simulink model "untitled"  (R2019a)
settings: Solver=VariableStepAuto  StartTime=0.0  StopTime=1  RelTol=1e-3
values from neighbouring files (symbols this model uses):
  Ts_Control = 5.0000e-05    (= 5e-05)    [Sec_Impedance.m]
  Ts_Power = 5.0000e-05    (= 5e-05)    [Sec_Impedance.m]
undefined symbols (not defined in the file or in its folder): D1, Delta, Ion, Lithium
libraries: powerlib x152, powerlib_meascontrol x65, simulink x14, electricdrivelib x12, simulink_extras x12
(part 1 of 5)
settings Model: SimulationMode=accelerator  Creator=ASUS  LastModifiedBy=ASUS

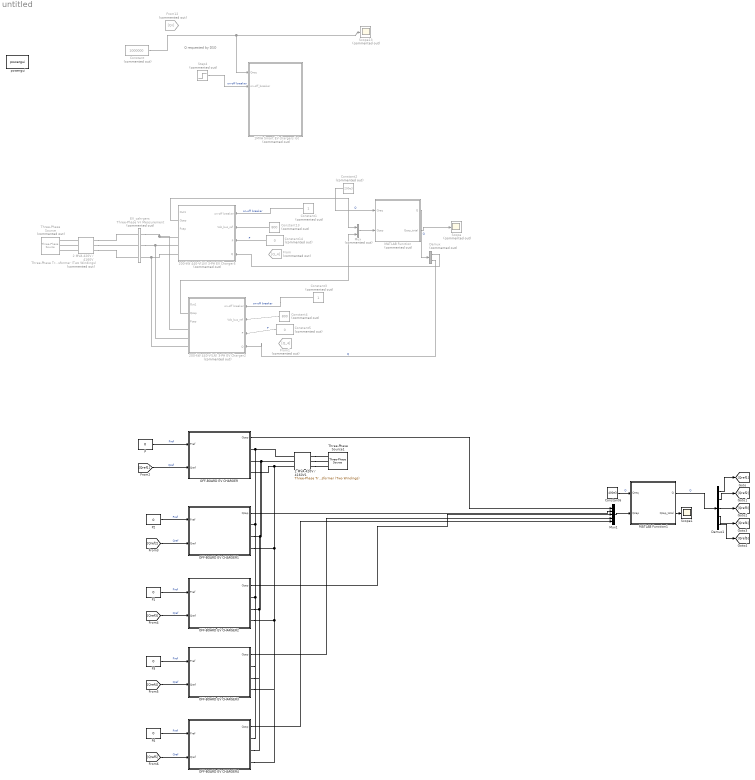
== system untitled ==
  note: Q requested by DSO
  1MVA Smart EV chargers lot : Subsystem  Commented=on
  2 MVA 420V / 4160V : powerlib/Elements/Three-Phase Transformer (Two Windings)  Commented=on  Winding1Connection=Delta (D1)  Winding2Connection=Yg  CoreType=Three single-phase transformers  SetSaturation=off  Hysteresis=off  DataFile='hysteresis'  SetInitialFlux=off  Measurements=None  UNITS=pu  NominalPower=[5e6 , 60 ]  Winding1=[ 4160 , 0.001 , 0.03 ]  Winding2=[ 420 , 0.001 , 0.03 ]  Rm=500  Lm=500  L0=0.5  Saturation=[ 0,0 ; 0.0024,1.2 ; 1.0,1.52 ]  InitialFluxes=[0.79999 -0.79999 0.7]  BreakLoop=off  DiscreteSolver=Trapezoidal iterative  DataType=off  TransfoNumber=0
      settings: SourceProductName=Simscape Electrical
  2 MVA 420V / 4160V1 : powerlib/Elements/Three-Phase Transformer (Two Windings)  Winding1Connection=Delta (D1)  Winding2Connection=Yg  CoreType=Three single-phase transformers  SetSaturation=off  Hysteresis=off  DataFile='hysteresis'  SetInitialFlux=off  Measurements=None  UNITS=pu  NominalPower=[5e6 , 60 ]  Winding1=[ 4160 , 0.001 , 0.03 ]  Winding2=[ 420 , 0.001 , 0.03 ]  Rm=500  Lm=500  L0=0.5  Saturation=[ 0,0 ; 0.0024,1.2 ; 1.0,1.52 ]  InitialFluxes=[0.79999 -0.79999 0.7]  BreakLoop=off  DiscreteSolver=Trapezoidal iterative  DataType=off  TransfoNumber=0
      settings: SourceProductName=Simscape Electrical
  200-kW 440-V(LN) 3-PH EV Charger2 : Subsystem  Commented=on
  200-kW 440-V(LN) 3-PH EV Charger5 : Subsystem  Commented=on
  Constant : Constant  Commented=on  Value=1000000
  Constant1 : Constant  Commented=on
  Constant13 : Constant  Commented=on  Value=800
  Constant14 : Constant  Commented=on  Value=0
  Constant2 : Constant  Commented=on  Value=200e3
  Constant3 : Constant  Commented=on
  Constant4 : Constant  Commented=on  Value=800
  Constant5 : Constant  Commented=on  Value=0
  Constant6 : Constant  Value=400e3
  Demux : Demux  Commented=on  Outputs=2
  Demux1 : Demux  Outputs=5
  EV_cahrgers : powerlib/Measurements/Three-Phase V-I Measurement  Commented=on  VoltageMeasurement=phase-to-ground  SetLabelV=on  LabelV=V_EV_cahrgers  Vpu=off  VpuLL=off  CurrentMeasurement=yes  SetLabelI=on  LabelI=I_EV_cahrgers  Ipu=off  Pbase=100e6  Vbase=500e3  OutputType=Magnitude  PhasorSimulation=off  PSBequivalent=0
      settings: SourceProductName=Simscape Electrical
  From : From  Commented=on  GotoTag=Q_4
  From1 : From  Commented=on  GotoTag=Q_4
  From12 : From  Commented=on  GotoTag=Qr
  MATLAB Function : MATLAB Function  Commented=on  TreatAsAtomicUnit=on
  MATLAB Function1 : MATLAB Function  TreatAsAtomicUnit=on
  Mux : Mux  Commented=on  Inputs=2
  Mux1 : Mux  Inputs=5
  OFF-BOARD EV CHARGER : Subsystem  mask(Off-board charger for EVs){Kp=1, Ki=20, C=3600e-6, Vdc=800, Ts=5e-5}
      mask prompts: Kp "Current Controller Kp"; Ki "Current Controller Ki"; C "DC link capacitor [uF]"; Vdc "DC link voltage level [V]"; Ts "Sample period [s]"
      mask help: This model only contains the three phase inverter and current controllers in rotating reference frame (PQ). The DAB converter need to be completed. It only has the inverter to improve the simulation time.
      mask Display: image('parking_lot3.png');
  OFF-BOARD EV CHARGER1 : Subsystem  mask(Off-board charger for EVs){Kp=1, Ki=20, C=3600e-6, Vdc=800, Ts=5e-5}
      mask prompts: Kp "Current Controller Kp"; Ki "Current Controller Ki"; C "DC link capacitor [uF]"; Vdc "DC link voltage level [V]"; Ts "Sample period [s]"
      mask help: This model only contains the three phase inverter and current controllers in rotating reference frame (PQ). The DAB converter need to be completed. It only has the inverter to improve the simulation time.
      mask Display: image('parking_lot3.png');
  OFF-BOARD EV CHARGER2 : Subsystem  mask(Off-board charger for EVs){Kp=1, Ki=20, C=3600e-6, Vdc=800, Ts=5e-5}
      mask prompts: Kp "Current Controller Kp"; Ki "Current Controller Ki"; C "DC link capacitor [uF]"; Vdc "DC link voltage level [V]"; Ts "Sample period [s]"
      mask help: This model only contains the three phase inverter and current controllers in rotating reference frame (PQ). The DAB converter need to be completed. It only has the inverter to improve the simulation time.
      mask Display: image('parking_lot3.png');
  OFF-BOARD EV CHARGER3 : Subsystem  mask(Off-board charger for EVs){Kp=1, Ki=20, C=3600e-6, Vdc=800, Ts=5e-5}
      mask prompts: Kp "Current Controller Kp"; Ki "Current Controller Ki"; C "DC link capacitor [uF]"; Vdc "DC link voltage level [V]"; Ts "Sample period [s]"
      mask help: This model only contains the three phase inverter and current controllers in rotating reference frame (PQ). The DAB converter need to be completed. It only has the inverter to improve the simulation time.
      mask Display: image('parking_lot3.png');
  OFF-BOARD EV CHARGER4 : Subsystem  mask(Off-board charger for EVs){Kp=1, Ki=20, C=3600e-6, Vdc=800, Ts=5e-5}
      mask prompts: Kp "Current Controller Kp"; Ki "Current Controller Ki"; C "DC link capacitor [uF]"; Vdc "DC link voltage level [V]"; Ts "Sample period [s]"
      mask help: This model only contains the three phase inverter and current controllers in rotating reference frame (PQ). The DAB converter need to be completed. It only has the inverter to improve the simulation time.
      mask Display: image('parking_lot3.png');
  P{,1..4} (5 alike) : Constant  Value=0
  Scope : Scope  Commented=on
  Scope1 : Scope
  Scope13 : Scope  Commented=on
  Step4 : Step  Commented=on  Time=0  SampleTime=0
  Three-Phase Source : powerlib/Electrical Sources/Three-Phase Source  Commented=on  InternalConnection=Yg  VoltagePhases=off  Voltage=4160  PhaseAngle=0  Voltage_phases=[25e3 25e3 25e3]/sqrt(3)  PhaseAngles_phases=[0 -120 +120]  Frequency=60  NonIdealSource=off  SpecifyImpedance=off  Resistance=0.8929  Inductance=16.58e-3  ShortCircuitLevel=100e6  BaseVoltage=25e3  XRratio=7  BusType=swing  Pref=10e3  Qref=0  Prefabc=[10e3, 10e3, 10e3]  Qrefabc=[0, 0, 0]  Qmin=-inf  Qmax=inf
      settings: SourceProductName=Simscape Electrical
  Three-Phase Source1 : powerlib/Electrical Sources/Three-Phase Source  InternalConnection=Yg  VoltagePhases=off  Voltage=4160  PhaseAngle=0  Voltage_phases=[25e3 25e3 25e3]/sqrt(3)  PhaseAngles_phases=[0 -120 +120]  Frequency=60  NonIdealSource=off  SpecifyImpedance=off  Resistance=0.8929  Inductance=16.58e-3  ShortCircuitLevel=100e6  BaseVoltage=25e3  XRratio=7  BusType=swing  Pref=10e3  Qref=0  Prefabc=[10e3, 10e3, 10e3]  Qrefabc=[0, 0, 0]  Qmin=-inf  Qmax=inf
      settings: SourceProductName=Simscape Electrical
  powergui : powerlib/powergui  Priority=1  SimulationMode=Discrete  SampleTime=50e-6  frequency=60  Iterations=50  frequencyindice=0  Pbase=100e6  ErrMax=0.0001  UnitsV=kV  UnitsW=MW  buscounter=0  FunctionMessages=off  echomessages=off  EnableUseOfTLC=off  CurrentSourceSwitches=off  DisableSnubberDevices=off  DisableRonSwitches=off  DisableVfSwitches=off  DisplayEquations=off  AutomaticDiscreteSolvers=off  SolverType=Tustin/Backward Euler (TBE)  Interpol=off  ExternalGateDelay=off  methode=off  Ts=0  x0status=blocks  SPID=off  SwTol=0  HookPort=off  NonlinearTolerance=0  nMaxIteration=15  ContinueOnMaxIteration=off  RestoreLinks=warning  ResistiveCurrentMeasurement=off  Frange=[0:2:500]  Ylog=off  Xlog=on  ShowGrid=off  save=off  variable=ZData  structure=0  ZoomFFT=off  StartTime=0.0  cycles=1  DisplayStyle=1  fundamental=60  FreqAxis=off  MaxFrequency=1000  frequencyindicesteady=1  RmsSteady=1  display=off
      settings: SourceProductName=Simscape Electrical
  wires:
  Step4/1 -> 1MVA Smart EV chargers lot/2(on-off_breaker)  "on-off breaker"
  Constant/1 -> 1MVA Smart EV chargers lot/1(Qreq), Scope13/1
  Constant1/1 -> 200-kW 440-V(LN) 3-PH EV Charger5/1(on-off breaker)  "on-off breaker"
  MATLAB Function/1(Q) -> Demux/1  "Q"
  Constant13/1 -> 200-kW 440-V(LN) 3-PH EV Charger5/2(Vdc_bus_ref)
  Constant14/1 -> 200-kW 440-V(LN) 3-PH EV Charger5/3(P)  "P"
  200-kW 440-V(LN) 3-PH EV Charger5/2(Qcap) -> Mux/1
  Constant2/1 -> MATLAB Function/1(Qreq)  "Q"
  MATLAB Function/2(Qcap_total) -> Scope/1
  Constant3/1 -> 200-kW 440-V(LN) 3-PH EV Charger2/1(on-off breaker)  "on-off breaker"
  Constant4/1 -> 200-kW 440-V(LN) 3-PH EV Charger2/2(Vdc_bus_ref)
  Constant5/1 -> 200-kW 440-V(LN) 3-PH EV Charger2/3(P)  "P"
  200-kW 440-V(LN) 3-PH EV Charger2/2(Qcap) -> Mux/2
  Demux/2 -> 200-kW 440-V(LN) 3-PH EV Charger2/4(Q)  "Q"
  Mux/1 -> MATLAB Function/2(Qcap)
  Demux/1 -> 200-kW 440-V(LN) 3-PH EV Charger5/4(Q)
  P/1 -> OFF-BOARD EV CHARGER/1(Pref)  "Pref"
  [Qref1] -> OFF-BOARD EV CHARGER/2(Qref)  "Qref"
  P2/1 -> OFF-BOARD EV CHARGER1/1(Pref)  "Pref"
  [Qref2] -> OFF-BOARD EV CHARGER1/2(Qref)  "Qref"
  MATLAB Function1/2(Qcap_total) -> Scope1/1
  Constant6/1 -> MATLAB Function1/1(Qreq)  "Q"
  OFF-BOARD EV CHARGER1/1(Qcap) -> Mux1/2
  MATLAB Function1/1(Q) -> Demux1/1  "Q"
  Mux1/1 -> MATLAB Function1/2(Qcap)
  OFF-BOARD EV CHARGER/1(Qcap) -> Mux1/1
  Demux1/1 -> [Qref1]
  Demux1/2 -> [Qref2]
  P1/1 -> OFF-BOARD EV CHARGER2/1(Pref)  "Pref"
  OFF-BOARD EV CHARGER2/1(Qcap) -> Mux1/3
  [Qref3] -> OFF-BOARD EV CHARGER2/2(Qref)  "Qref"
  P3/1 -> OFF-BOARD EV CHARGER3/1(Pref)  "Pref"
  [Qref4] -> OFF-BOARD EV CHARGER3/2(Qref)  "Qref"
  P4/1 -> OFF-BOARD EV CHARGER4/1(Pref)  "Pref"
  [Qref5] -> OFF-BOARD EV CHARGER4/2(Qref)  "Qref"
  Demux1/3 -> [Qref3]
  Demux1/4 -> [Qref4]
  Demux1/5 -> [Qref5]
  OFF-BOARD EV CHARGER3/1(Qcap) -> Mux1/4
  OFF-BOARD EV CHARGER4/1(Qcap) -> Mux1/5
  connections:
  EV_cahrgers/LConn2 -- 200-kW 440-V(LN) 3-PH EV Charger2/RConn2 -- 200-kW 440-V(LN) 3-PH EV Charger5/RConn2
  200-kW 440-V(LN) 3-PH EV Charger5/RConn3 -- 200-kW 440-V(LN) 3-PH EV Charger2/RConn3 -- EV_cahrgers/LConn3
  2 MVA 420V / 4160V/RConn1 -- EV_cahrgers/RConn1
  2 MVA 420V / 4160V/RConn3 -- EV_cahrgers/RConn3
  EV_cahrgers/LConn1 -- 200-kW 440-V(LN) 3-PH EV Charger2/RConn1 -- 200-kW 440-V(LN) 3-PH EV Charger5/RConn1
  2 MVA 420V / 4160V/RConn2 -- EV_cahrgers/RConn2
  2 MVA 420V / 4160V/LConn1 -- Three-Phase Source/RConn1
  2 MVA 420V / 4160V/LConn2 -- Three-Phase Source/RConn2
  2 MVA 420V / 4160V/LConn3 -- Three-Phase Source/RConn3
  2 MVA 420V / 4160V1/LConn1 -- Three-Phase Source1/RConn1
  2 MVA 420V / 4160V1/LConn2 -- Three-Phase Source1/RConn2
  2 MVA 420V / 4160V1/RConn1 -- OFF-BOARD EV CHARGER4/RConn1 -- OFF-BOARD EV CHARGER3/RConn1 -- OFF-BOARD EV CHARGER2/RConn1 -- OFF-BOARD EV CHARGER1/RConn1 -- OFF-BOARD EV CHARGER/RConn1
  2 MVA 420V / 4160V1/LConn3 -- Three-Phase Source1/RConn3
  2 MVA 420V / 4160V1/RConn2 -- OFF-BOARD EV CHARGER4/RConn2 -- OFF-BOARD EV CHARGER3/RConn2 -- OFF-BOARD EV CHARGER2/RConn2 -- OFF-BOARD EV CHARGER1/RConn2 -- OFF-BOARD EV CHARGER/RConn2
  2 MVA 420V / 4160V1/RConn3 -- OFF-BOARD EV CHARGER4/RConn3 -- OFF-BOARD EV CHARGER3/RConn3 -- OFF-BOARD EV CHARGER2/RConn3 -- OFF-BOARD EV CHARGER1/RConn3 -- OFF-BOARD EV CHARGER/RConn3

== system untitled/1MVA Smart EV chargers lot ==
  note: Q requested by DSO
  note: Smart EV chargers lot
  note: AGGREGATOR
  Qreq : Inport
  on-off_breaker : Inport  Port=2
  200-kW 440-V(LN) 3-PH EV Charger : Subsystem
  200-kW 440-V(LN) 3-PH EV Charger2 : Subsystem
  200-kW 440-V(LN) 3-PH EV Charger3 : Subsystem
  200-kW 440-V(LN) 3-PH EV Charger4 : Subsystem
  200-kW 440-V(LN) 3-PH EV Charger5 : Subsystem
  Constant{,2,6,8,14} (5 alike) : Constant  Value=0
  Constant{3,5,9,11,13} (5 alike) : Constant  Value=800
  Demux : Demux  Outputs=5
  MATLAB Function : MATLAB Function  TreatAsAtomicUnit=on
  Mux : Mux  Inputs=5
  Scope{,2..6} (6 alike) : Scope
  a : PMIOPort  Side=Left
  b : PMIOPort  Port=2  Side=Left
  c : PMIOPort  Port=3  Side=Left
  wires:
  Constant14/1 -> 200-kW 440-V(LN) 3-PH EV Charger5/3(P)  "P"
  200-kW 440-V(LN) 3-PH EV Charger4/1(Out1) -> Scope5/1
  [Q_1] -> 200-kW 440-V(LN) 3-PH EV Charger/4(Q)  "Q"
  Constant11/1 -> 200-kW 440-V(LN) 3-PH EV Charger4/2(Vdc_bus_ref)
  Constant/1 -> 200-kW 440-V(LN) 3-PH EV Charger/3(P)  "P"
  [Q_3] -> 200-kW 440-V(LN) 3-PH EV Charger3/4(Q)  "Q"
  on-off_breaker/1 -> 200-kW 440-V(LN) 3-PH EV Charger5/1(on-off breaker), 200-kW 440-V(LN) 3-PH EV Charger4/1(on-off breaker), 200-kW 440-V(LN) 3-PH EV Charger2/1(on-off breaker), 200-kW 440-V(LN) 3-PH EV Charger/1(on-off breaker), 200-kW 440-V(LN) 3-PH EV Charger3/1(on-off breaker)  "on-off breaker"
  [Q_2] -> 200-kW 440-V(LN) 3-PH EV Charger2/4(Q)  "Q"
  Constant2/1 -> 200-kW 440-V(LN) 3-PH EV Charger2/3(P)  "P"
  Constant3/1 -> 200-kW 440-V(LN) 3-PH EV Charger/2(Vdc_bus_ref)
  [Q_5] -> 200-kW 440-V(LN) 3-PH EV Charger4/4(Q)  "Q"
  200-kW 440-V(LN) 3-PH EV Charger/1(Out1) -> Scope2/1
  Constant8/1 -> 200-kW 440-V(LN) 3-PH EV Charger4/3(P)  "P"
  200-kW 440-V(LN) 3-PH EV Charger2/1(Out1) -> Scope3/1
  Constant13/1 -> 200-kW 440-V(LN) 3-PH EV Charger5/2(Vdc_bus_ref)
  200-kW 440-V(LN) 3-PH EV Charger5/1(Out1) -> Scope6/1
  [Q_4] -> 200-kW 440-V(LN) 3-PH EV Charger5/4(Q)  "Q"
  Constant6/1 -> 200-kW 440-V(LN) 3-PH EV Charger3/3(P)  "P"
  Constant9/1 -> 200-kW 440-V(LN) 3-PH EV Charger3/2(Vdc_bus_ref)
  200-kW 440-V(LN) 3-PH EV Charger3/1(Out1) -> Scope4/1
  Constant5/1 -> 200-kW 440-V(LN) 3-PH EV Charger2/2(Vdc_bus_ref)
  Qreq/1 -> MATLAB Function/1(Qreq)
  200-kW 440-V(LN) 3-PH EV Charger5/2(Qcap) -> Mux/5
  200-kW 440-V(LN) 3-PH EV Charger4/2(Qcap) -> Mux/4
  Mux/1 -> MATLAB Function/2(Qcap)
  200-kW 440-V(LN) 3-PH EV Charger3/2(Qcap) -> Mux/3
  200-kW 440-V(LN) 3-PH EV Charger2/2(Qcap) -> Mux/2
  200-kW 440-V(LN) 3-PH EV Charger/2(Qcap) -> Mux/1
  MATLAB Function/2(Qcap_total) -> Scope/1
  MATLAB Function/1(Q) -> Demux/1
  Demux/1 -> [Q_1]
  Demux/3 -> [Q_3]
  Demux/5 -> [Q_5]
  Demux/4 -> [Q_4]
  Demux/2 -> [Q_2]
  connections:
  200-kW 440-V(LN) 3-PH EV Charger4/RConn1 -- 200-kW 440-V(LN) 3-PH EV Charger5/RConn1 -- 200-kW 440-V(LN) 3-PH EV Charger3/RConn1 -- 200-kW 440-V(LN) 3-PH EV Charger2/RConn1 -- a/RConn1 -- 200-kW 440-V(LN) 3-PH EV Charger/RConn1
  200-kW 440-V(LN) 3-PH EV Charger4/RConn3 -- 200-kW 440-V(LN) 3-PH EV Charger5/RConn3 -- 200-kW 440-V(LN) 3-PH EV Charger2/RConn3 -- c/RConn1 -- 200-kW 440-V(LN) 3-PH EV Charger/RConn3 -- 200-kW 440-V(LN) 3-PH EV Charger3/RConn3
  200-kW 440-V(LN) 3-PH EV Charger4/RConn2 -- 200-kW 440-V(LN) 3-PH EV Charger5/RConn2 -- 200-kW 440-V(LN) 3-PH EV Charger3/RConn2 -- 200-kW 440-V(LN) 3-PH EV Charger2/RConn2 -- b/RConn1 -- 200-kW 440-V(LN) 3-PH EV Charger/RConn2

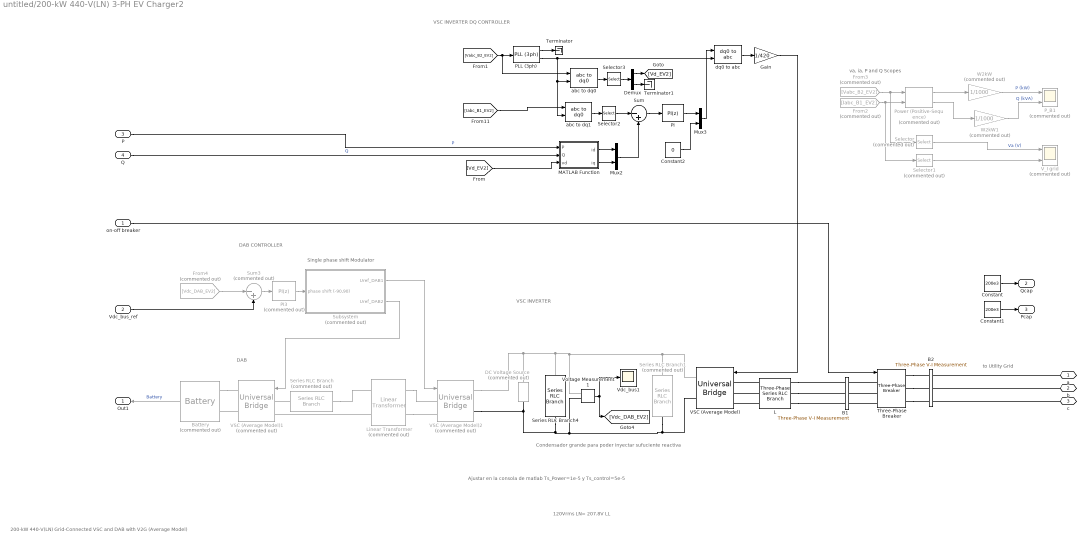
== system untitled/200-kW 440-V(LN) 3-PH EV Charger2 ==
  note: DAB CONTROLLER
  note: va, ia, P and Q Scopes
  note: 200-kW 440-V(LN) Grid-Connected VSC and DAB with V2G (Average Model)
  note: 120Vrms LN= 207.8V LL
  note: Single phase shift Modulator
  note: Condensador grande para poder inyectar sufuciente reactiva
  note: Ajustar en la consola de matlab Ts_Power=1e-5 y Ts_control=5e-5
  note: to Utility Grid
  note: DAB
  note: VSC INVERTER
  note: VSC INVERTER DQ CONTROLLER
  on-off breaker : Inport
  Vdc_bus_ref : Inport  Port=2
  P : Inport  Port=3
  Q : Inport  Port=4
  B1 : powerlib/Measurements/Three-Phase V-I Measurement  VoltageMeasurement=no  SetLabelV=on  LabelV=Vabc_B1  Vpu=off  VpuLL=off  CurrentMeasurement=yes  SetLabelI=on  LabelI=Iabc_B1_EV2  Ipu=off  Pbase=100e6  Vbase=500e3  OutputType=Magnitude  PhasorSimulation=off  PSBequivalent=0
      settings: SourceProductName=Simscape Electrical
  B2 : powerlib/Measurements/Three-Phase V-I Measurement  VoltageMeasurement=phase-to-ground  SetLabelV=on  LabelV=Vabc_B2_EV2  Vpu=off  VpuLL=off  CurrentMeasurement=no  SetLabelI=off  LabelI=Iabc_B1  Ipu=off  Pbase=100e6  Vbase=500e3  OutputType=Magnitude  PhasorSimulation=off  PSBequivalent=0
      settings: SourceProductName=Simscape Electrical
  Battery : electricdrivelib/Extra Sources/Battery  Commented=on  BatType=Lithium-Ion  ShowTempParam=off  ThermalPreset=no  ShowAgeParam=off  NomV=380  NomQ=5.4*70  SOC=70  Batt_Tr=20  PresetModel=on  MaxQ=378  MinV=285  FullV=442.3151  Dis_rate=164.3478  R=0.010053  Normal_OP=341.8435  expZone="[410.5466       18.5713]"  current=[6.5 13 32.5]  Units=Time  Tci=20  NomT=20  T2=-30  MaxQ2=4.8  FullV2=7.1  Normal_OP2=5.655  expZone2="[6.58           1]"  Rca=0.6  ti=2000  Dp=0  Neq0=0  Tsim=1e6  Ta1=25  Qeol=5.4*0.9  Reol=0.013333*1.2  Char_age=[2.3478, 3]  Dis_age=[2.3478, 10]  N1=1500  N2=10500  N3=1000  N4=1400  Ta2=45  N5=950
      settings: SourceProductName=Simscape Electrical
  Constant : Constant  Value=200e3
  Constant1 : Constant  Value=200e3
  Constant2 : Constant  Value=0
  DC Voltage Source : powerlib/Electrical Sources/DC Voltage Source  Commented=on  Amplitude=800  Measurements=None
      settings: SourceProductName=Simscape Electrical
  Demux : Demux  Outputs=2
  From2 : From  Commented=on  GotoTag=Iabc_B1_EV2  TagVisibility=global
      settings: CloseFcn=tagdialog Close
  From3 : From  Commented=on  GotoTag=Vabc_B2_EV2  TagVisibility=global
      settings: CloseFcn=tagdialog Close
  From4 : From  Commented=on  GotoTag=Vdc_DAB_EV2
  Gain : Gain  Gain=1/420
  L : powerlib/Elements/Three-Phase Series RLC Branch  LConnTagsString=A|B|C  RConnTagsString=A|B|C  BranchType=RL  Resistance=500e-6*377/50/2  Inductance=1200e-6/2  Capacitance=inf  Measurements=None
      settings: SourceProductName=Simscape Electrical
  Linear Transformer : powerlib/Elements/Linear Transformer  Commented=on  UNITS=SI  NominalPower=[ 250e3 10000 ]  winding1=[400 0.0032 0.4883e-06]  winding2=[800 0.0032 0.4883e-06]  ThreeWindings=off  winding3=[3.15e+05 19845 2105.6]  RmLm=[800 2.1221]  Measurements=None  DataType=on
      settings: SourceProductName=Simscape Electrical
  MATLAB Function : MATLAB Function  TreatAsAtomicUnit=on
  Mux2 : Mux  Inputs=2
  Mux3 : Mux  Inputs=2
  PI : simulink/Continuous/PID Controller  Controller=PI  Form=Parallel  TimeDomain=Discrete-time  SampleTime=Ts_Control  IntegratorMethod=Forward Euler  FilterMethod=Forward Euler  ControllerParametersSource=internal  P=20  I=360  D=0  UseFilter=on  N=100  TunerSelectOption=Transfer Function Based (PID Tuner App)  InitialConditionSource=internal  InitialConditionForIntegrator=0  InitialConditionForFilter=0  DifferentiatorICPrevScaledInput=0  ExternalReset=none  TrackingMode=off  Kt=1  LimitOutput=on  UpperSaturationLimit=800  LowerSaturationLimit=-800  LinearizeAsGain=off  AntiWindupMode=none  Kb=1  POutMin=[]  POutMax=[]  IOutMin=[]  IOutMax=[]  DOutMin=[]  DOutMax=[]  NOutMin=[]  NOutMax=[]  SumOutMin=[]  SumOutMax=[]  SaturationOutMin=[]  SaturationOutMax=[]  PParamMin=[]  PParamMax=[]  IParamMin=[]  IParamMax=[]  DParamMin=[]  DParamMax=[]  NParamMin=[]  NParamMax=[]  KbParamMin=[]  KbParamMax=[]  KtParamMin=[]  KtParamMax=[]  KbOutMin=[]  KbOutMax=[]  KtOutMin=[]  KtOutMax=[]  IntegratorOutMin=[]  IntegratorOutMax=[]  FilterOutMin=[]  FilterOutMax=[]  SumI1OutMin=[]  SumI1OutMax=[]  SumI2OutMin=[]  SumI2OutMax=[]  SumI3OutMin=[]  SumI3OutMax=[]  SumI4OutMin=[]  SumI4OutMax=[]  SumDOutMin=[]  SumDOutMax=[]  DifferentiatorOutMin=[]  DifferentiatorOutMax=[]  FilterDiffOutCoefMin=[]  FilterDiffOutCoefMax=[]  ReciprocalOutMin=[]  ReciprocalOutMax=[]  SumDenOutMin=[]  SumDenOutMax=[]  SumNumOutMin=[]  SumNumOutMax=[]  DivideOutMin=[]  DivideOutMax=[]  IntegratorContinuousStateAttributes=''  IntegratorStateMustResolveToSignalObject=off  IntegratorRTWStateStorageClass=Auto  FilterContinuousStateAttributes=''  FilterStateMustResolveToSignalObject=off  FilterRTWStateStorageClass=Auto  ParallelPVariant=InternalParameters  IdealPVariant=Disabled  IVariant=InternalParameters  DVariant=Disabled  IntegratorVariant=Discrete  SatVariant=Enabled  AWVariant=Passthrough  PCopyVariant=Disabled  TRVariant=Disabled  FdbkBlocksVariant=Forward  IdealPFdbkVariant=Disabled  SatFdbkVariant=Disabled  DerivativeFilterVariant=Disabled  NVariant=Disabled  NCopyVariant=Disabled_SignalSpec  FilterICVariant=Disabled  IntegratorICVariant=InternalICs  ExternalResetVariant=Disabled  TRSumVariant=Passthrough  SumFdbkVariant=Disabled  SumVariant=Sum_PI
  PI3 : simulink/Continuous/PID Controller  Commented=on  Controller=PI  Form=Parallel  TimeDomain=Discrete-time  SampleTime=Ts_Control  IntegratorMethod=Forward Euler  FilterMethod=Forward Euler  ControllerParametersSource=internal  P=4  I=50  D=0  UseFilter=on  N=100  TunerSelectOption=Transfer Function Based (PID Tuner App)  InitialConditionSource=internal  InitialConditionForIntegrator=0  InitialConditionForFilter=0  DifferentiatorICPrevScaledInput=0  ExternalReset=none  TrackingMode=off  Kt=1  LimitOutput=on  UpperSaturationLimit=90  LowerSaturationLimit=-90  LinearizeAsGain=off  AntiWindupMode=none  Kb=1  POutMin=[]  POutMax=[]  IOutMin=[]  IOutMax=[]  DOutMin=[]  DOutMax=[]  NOutMin=[]  NOutMax=[]  SumOutMin=[]  SumOutMax=[]  SaturationOutMin=[]  SaturationOutMax=[]  PParamMin=[]  PParamMax=[]  IParamMin=[]  IParamMax=[]  DParamMin=[]  DParamMax=[]  NParamMin=[]  NParamMax=[]  KbParamMin=[]  KbParamMax=[]  KtParamMin=[]  KtParamMax=[]  KbOutMin=[]  KbOutMax=[]  KtOutMin=[]  KtOutMax=[]  IntegratorOutMin=[]  IntegratorOutMax=[]  FilterOutMin=[]  FilterOutMax=[]  SumI1OutMin=[]  SumI1OutMax=[]  SumI2OutMin=[]  SumI2OutMax=[]  SumI3OutMin=[]  SumI3OutMax=[]  SumI4OutMin=[]  SumI4OutMax=[]  SumDOutMin=[]  SumDOutMax=[]  DifferentiatorOutMin=[]  DifferentiatorOutMax=[]  FilterDiffOutCoefMin=[]  FilterDiffOutCoefMax=[]  ReciprocalOutMin=[]  ReciprocalOutMax=[]  SumDenOutMin=[]  SumDenOutMax=[]  SumNumOutMin=[]  SumNumOutMax=[]  DivideOutMin=[]  DivideOutMax=[]  IntegratorContinuousStateAttributes=''  IntegratorStateMustResolveToSignalObject=off  IntegratorRTWStateStorageClass=Auto  FilterContinuousStateAttributes=''  FilterStateMustResolveToSignalObject=off  FilterRTWStateStorageClass=Auto  ParallelPVariant=InternalParameters  IdealPVariant=Disabled  IVariant=InternalParameters  DVariant=Disabled  IntegratorVariant=Discrete  SatVariant=Enabled  AWVariant=Passthrough  PCopyVariant=Disabled  TRVariant=Disabled  FdbkBlocksVariant=Forward  IdealPFdbkVariant=Disabled  SatFdbkVariant=Disabled  DerivativeFilterVariant=Disabled  NVariant=Disabled  NCopyVariant=Disabled_SignalSpec  FilterICVariant=Disabled  IntegratorICVariant=InternalICs  ExternalResetVariant=Disabled  TRSumVariant=Passthrough  SumFdbkVariant=Disabled  SumVariant=Sum_PI
  PLL (3ph) : powerlib_meascontrol/PLL/PLL (3ph)  Fmin=55  Par_Init="[-0.57  60]"  ParK=[180, 3200, 1]  TcD=1e-4  MaxRateChangeFreq=12  FilterCutOffFreq=25  Ts=Ts_Power  AGC=on
      settings: SourceProductName=Simscape Electrical
  P_B1 : Scope  Commented=on  NumInputPorts=2
  Power (Positive-Sequence) : powerlib_meascontrol/Measurements/Power (Positive-Sequence)  Commented=on  Freq=60  Vinit=[0, 0]  Iinit=[0, 0]  Ts=Ts_Control
      settings: SourceProductName=Simscape Electrical  SourceProductBaseCode=PS
  Selector : Selector  Commented=on  InputPortWidth=3  IndexOptions=Index vector (dialog)  Indices=[1]  OutputSizes=1
  Selector1 : Selector  Commented=on  InputPortWidth=3  IndexOptions=Index vector (dialog)  Indices=[1]  OutputSizes=1
  Selector2 : Selector  InputPortWidth=3  IndexOptions=Index vector (dialog)  Indices=[1 2]  OutputSizes=1
  Selector3 : Selector  InputPortWidth=3  IndexOptions=Index vector (dialog)  Indices=[1 2]  OutputSizes=1
  Series RLC Branch : powerlib/Elements/Series RLC Branch  Commented=on  LConnTagsString=__new0  RConnTagsString=__new0  BranchType=L  Resistance=1  Inductance=1.5e-6  SetiL0=off  InitialCurrent=0  Capacitance=1e-6  Setx0=off  InitialVoltage=0  Measurements=None
      settings: SourceProductName=Simscape Electrical
  Series RLC Branch1 : powerlib/Elements/Series RLC Branch  Commented=on  LConnTagsString=__new0  RConnTagsString=__new0  BranchType=R  Resistance=3.2  Inductance=1e-3  SetiL0=off  InitialCurrent=0  Capacitance=1200e-6  Setx0=off  InitialVoltage=400  Measurements=None
      settings: SourceProductName=Simscape Electrical
  Series RLC Branch4 : powerlib/Elements/Series RLC Branch  LConnTagsString=__new0  RConnTagsString=__new0  BranchType=RC  Resistance=1e-7  Inductance=1e-3  SetiL0=off  InitialCurrent=0  Capacitance=3600e-6  Setx0=off  InitialVoltage=400  Measurements=None
      settings: SourceProductName=Simscape Electrical
  Subsystem : Subsystem  Commented=on
  Sum : Sum  Inputs=|-+
  Sum3 : Sum  Commented=on  Inputs=|-+
  Terminator : Terminator
  Terminator1 : Terminator
  Three-Phase Breaker : powerlib/Elements/Three-Phase Breaker  InitialState=open  SwitchA=on  SwitchB=on  SwitchC=on  SwitchTimes="[1/6  5/6]"  External=on  BreakerResistance=0.01e-3  SnubberResistance=30  SnubberCapacitance=20e-6  Measurements=None
      settings: SourceProductName=Simscape Electrical
  VSC (Average Model) : powerlib/Power Electronics/Universal Bridge  Arms=3  SnubberResistance=1e5  SnubberCapacitance=inf  Device=Average-model based VSC  Ron=1e-3  Lon=0  ForwardVoltages="[  0  0  ]"  ForwardVoltage=0  GTOparameters=[ 10e-6 , 20e-6 ]  IGBTparameters=[ 1e-6 , 2e-6 ]  Measurements=None  Measurements_2=None  converterType=Rectifier
      settings: SourceProductName=Simscape Electrical
  VSC (Average Model)1 : powerlib/Power Electronics/Universal Bridge  Commented=on  Arms=2  SnubberResistance=1e5  SnubberCapacitance=inf  Device=Average-model based VSC  Ron=1e-3  Lon=0  ForwardVoltages="[  0  0  ]"  ForwardVoltage=0  GTOparameters=[ 10e-6 , 20e-6 ]  IGBTparameters=[ 1e-6 , 2e-6 ]  Measurements=None  Measurements_2=None  converterType=Rectifier
      settings: SourceProductName=Simscape Electrical
  VSC (Average Model)2 : powerlib/Power Electronics/Universal Bridge  Commented=on  Arms=2  SnubberResistance=1e5  SnubberCapacitance=inf  Device=Average-model based VSC  Ron=1e-3  Lon=0  ForwardVoltages="[  0  0  ]"  ForwardVoltage=0  GTOparameters=[ 10e-6 , 20e-6 ]  IGBTparameters=[ 1e-6 , 2e-6 ]  Measurements=None  Measurements_2=None  converterType=Rectifier
      settings: SourceProductName=Simscape Electrical
  V_I grid : Scope  Commented=on  NumInputPorts=2
  Vdc_bus1 : Scope
  Voltage Measurement1 : powerlib/Measurements/Voltage Measurement  PhasorSimulation=off  OutputType=Complex  PSBequivalent=0
      settings: SourceProductName=Simscape Electrical
  W2kW : Gain  Commented=on  Gain=1/1000
  W2kW1 : Gain  Commented=on  Gain=1/1000
  abc to dq0 : powerlib_meascontrol/Transformations/abc to dq0  Alignment=90 degrees behind phase A axis
      settings: SourceProductName=Simscape Electrical
  abc to dq1 : powerlib_meascontrol/Transformations/abc to dq0  Alignment=90 degrees behind phase A axis
      settings: SourceProductName=Simscape Electrical
  dq0 to abc : powerlib_meascontrol/Transformations/dq0 to abc  Alignment=90 degrees behind phase A axis
      settings: SourceProductName=Simscape Electrical
  a : PMIOPort  Side=Right
  b : PMIOPort  Port=2  Side=Right
  c : PMIOPort  Port=3  Side=Right
  Out1 : Outport
  Qcap : Outport  Port=2
  Pcap : Outport  Port=3
  wires:
  PLL (3ph)/2 -> abc to dq1/2, abc to dq0/2, dq0 to abc/2
  Subsystem/1(Uref_DAB1) -> VSC (Average Model)2/1
  PI/1 -> Mux3/1
  Selector/1 -> V_I grid/1  "Va (V)"
  dq0 to abc/1 -> Gain/1
  Vdc_bus_ref/1 -> Sum3/2
  PLL (3ph)/1 -> Terminator/1
  From2/1 -> Selector1/1, Power (Positive-Sequence)/2
  abc to dq1/1 -> Selector2/1
  Mux3/1 -> dq0 to abc/1
  Gain/1 -> VSC (Average Model)/1
  W2kW1/1 -> P_B1/2  "Q (kVA)"
  Selector2/1 -> Sum/1
  Sum/1 -> PI/1
  [Vabc_B2_EV2] -> abc to dq0/1, PLL (3ph)/1
  Subsystem/2(Uref_DAB2) -> VSC (Average Model)1/1
  Sum3/1 -> PI3/1
  W2kW/1 -> P_B1/1  "P (kW)"
  Constant2/1 -> Mux3/2
  PI3/1 -> Subsystem/1(phase shift (-90,90))
  Selector3/1 -> Demux/1
  From3/1 -> Selector/1, Power (Positive-Sequence)/1
  Selector1/1 -> V_I grid/2
  From4/1 -> Sum3/1
  abc to dq0/1 -> Selector3/1
  Power (Positive-Sequence)/1 -> W2kW/1
  Voltage Measurement1/1 -> Vdc_bus1/1, [Vdc_DAB_EV2]
  Mux2/1 -> Sum/2
  [Iabc_B1_EV2] -> abc to dq1/1
  Power (Positive-Sequence)/2 -> W2kW1/1
  Battery/1 -> Out1/1  "Battery"
  on-off breaker/1 -> Three-Phase Breaker/1
  Demux/2 -> Terminator1/1
  Demux/1 -> [Vd_EV2]
  MATLAB Function/1(id) -> Mux2/1
  MATLAB Function/2(iq) -> Mux2/2
  [Vd_EV2] -> MATLAB Function/3(vd)
  P/1 -> MATLAB Function/1(P)  "P"
  Q/1 -> MATLAB Function/2(Q)  "Q"
  Constant1/1 -> Pcap/1
  Constant/1 -> Qcap/1
  connections:
  Battery/LConn1 -- VSC (Average Model)1/RConn1
  Three-Phase Breaker/LConn1 -- B1/RConn1
  Three-Phase Breaker/RConn2 -- B2/LConn2
  VSC (Average Model)/RConn2 -- Series RLC Branch1/RConn1 -- VSC (Average Model)2/RConn2 -- DC Voltage Source/LConn1 -- Series RLC Branch4/RConn1 -- Voltage Measurement1/LConn2
  L/RConn3 -- B1/LConn3
  L/LConn1 -- VSC (Average Model)/LConn1
  L/RConn1 -- B1/LConn1
  L/LConn2 -- VSC (Average Model)/LConn2
  Series RLC Branch1/LConn1 -- VSC (Average Model)/RConn1 -- DC Voltage Source/RConn1 -- VSC (Average Model)2/RConn1 -- Series RLC Branch4/LConn1 -- Voltage Measurement1/LConn1
  Series RLC Branch/RConn1 -- Linear Transformer/LConn1
  Linear Transformer/LConn2 -- VSC (Average Model)1/LConn2
  Three-Phase Breaker/LConn2 -- B1/RConn2
  VSC (Average Model)1/RConn2 -- Battery/LConn2
  Three-Phase Breaker/RConn3 -- B2/LConn3
  Three-Phase Breaker/RConn1 -- B2/LConn1
  Linear Transformer/RConn1 -- VSC (Average Model)2/LConn1
  Linear Transformer/RConn2 -- VSC (Average Model)2/LConn2
  c/RConn1 -- B2/RConn3
  Series RLC Branch/LConn1 -- VSC (Average Model)1/LConn1
  L/RConn2 -- B1/LConn2
  L/LConn3 -- VSC (Average Model)/LConn3
  Three-Phase Breaker/LConn3 -- B1/RConn3
  b/RConn1 -- B2/RConn2
  a/RConn1 -- B2/RConn1

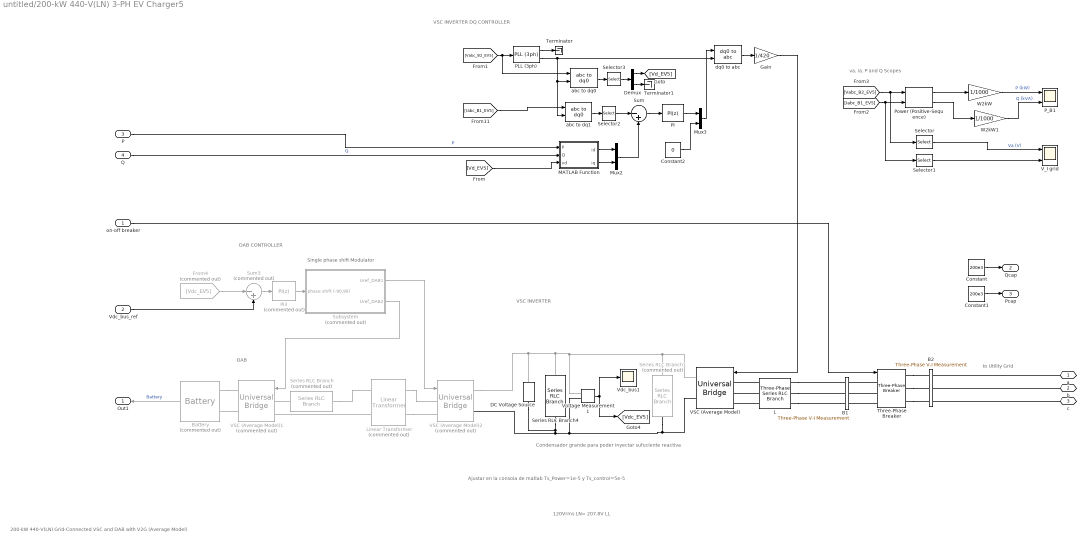
== system untitled/200-kW 440-V(LN) 3-PH EV Charger5 ==
  note: DAB CONTROLLER
  note: va, ia, P and Q Scopes
  note: 200-kW 440-V(LN) Grid-Connected VSC and DAB with V2G (Average Model)
  note: 120Vrms LN= 207.8V LL
  note: Single phase shift Modulator
  note: Condensador grande para poder inyectar sufuciente reactiva
  note: Ajustar en la consola de matlab Ts_Power=1e-5 y Ts_control=5e-5
  note: to Utility Grid
  note: DAB
  note: VSC INVERTER
  note: VSC INVERTER DQ CONTROLLER
  on-off breaker : Inport
  Vdc_bus_ref : Inport  Port=2
  P : Inport  Port=3
  Q : Inport  Port=4
  B1 : powerlib/Measurements/Three-Phase V-I Measurement  VoltageMeasurement=no  SetLabelV=on  LabelV=Vabc_B1  Vpu=off  VpuLL=off  CurrentMeasurement=yes  SetLabelI=on  LabelI=Iabc_B1_EV5  Ipu=off  Pbase=100e6  Vbase=500e3  OutputType=Magnitude  PhasorSimulation=off  PSBequivalent=0
      settings: SourceProductName=Simscape Electrical
  B2 : powerlib/Measurements/Three-Phase V-I Measurement  VoltageMeasurement=phase-to-ground  SetLabelV=on  LabelV=Vabc_B2_EV5  Vpu=off  VpuLL=off  CurrentMeasurement=no  SetLabelI=off  LabelI=Iabc_B1  Ipu=off  Pbase=100e6  Vbase=500e3  OutputType=Magnitude  PhasorSimulation=off  PSBequivalent=0
      settings: SourceProductName=Simscape Electrical
  Battery : electricdrivelib/Extra Sources/Battery  Commented=on  BatType=Lithium-Ion  ShowTempParam=off  ThermalPreset=no  ShowAgeParam=off  NomV=380  NomQ=5.4*70  SOC=70  Batt_Tr=20  PresetModel=on  MaxQ=378  MinV=285  FullV=442.3151  Dis_rate=164.3478  R=0.010053  Normal_OP=341.8435  expZone="[410.5466       18.5713]"  current=[6.5 13 32.5]  Units=Time  Tci=20  NomT=20  T2=-30  MaxQ2=4.8  FullV2=7.1  Normal_OP2=5.655  expZone2="[6.58           1]"  Rca=0.6  ti=2000  Dp=0  Neq0=0  Tsim=1e6  Ta1=25  Qeol=5.4*0.9  Reol=0.013333*1.2  Char_age=[2.3478, 3]  Dis_age=[2.3478, 10]  N1=1500  N2=10500  N3=1000  N4=1400  Ta2=45  N5=950
      settings: SourceProductName=Simscape Electrical
  Constant : Constant  Value=200e3
  Constant1 : Constant  Value=200e3
  Constant2 : Constant  Value=0
  DC Voltage Source : powerlib/Electrical Sources/DC Voltage Source  Amplitude=800  Measurements=None
      settings: SourceProductName=Simscape Electrical
  Demux : Demux  Outputs=2
  From4 : From  Commented=on  GotoTag=Vdc_EV5
  Gain : Gain  Gain=1/420
  L : powerlib/Elements/Three-Phase Series RLC Branch  LConnTagsString=A|B|C  RConnTagsString=A|B|C  BranchType=RL  Resistance=500e-6*377/50/2  Inductance=1200e-6/2  Capacitance=inf  Measurements=None
      settings: SourceProductName=Simscape Electrical
  Linear Transformer : powerlib/Elements/Linear Transformer  Commented=on  UNITS=SI  NominalPower=[ 250e3 10000 ]  winding1=[400 0.0032 0.4883e-06]  winding2=[800 0.0032 0.4883e-06]  ThreeWindings=off  winding3=[3.15e+05 19845 2105.6]  RmLm=[800 2.1221]  Measurements=None  DataType=on
      settings: SourceProductName=Simscape Electrical
  MATLAB Function : MATLAB Function  TreatAsAtomicUnit=on
  Mux2 : Mux  Inputs=2
  Mux3 : Mux  Inputs=2
  PI : simulink/Continuous/PID Controller  Controller=PI  Form=Parallel  TimeDomain=Discrete-time  SampleTime=Ts_Control  IntegratorMethod=Forward Euler  FilterMethod=Forward Euler  ControllerParametersSource=internal  P=20  I=360  D=0  UseFilter=on  N=100  TunerSelectOption=Transfer Function Based (PID Tuner App)  InitialConditionSource=internal  InitialConditionForIntegrator=0  InitialConditionForFilter=0  DifferentiatorICPrevScaledInput=0  ExternalReset=none  TrackingMode=off  Kt=1  LimitOutput=on  UpperSaturationLimit=800  LowerSaturationLimit=-800  LinearizeAsGain=off  AntiWindupMode=none  Kb=1  POutMin=[]  POutMax=[]  IOutMin=[]  IOutMax=[]  DOutMin=[]  DOutMax=[]  NOutMin=[]  NOutMax=[]  SumOutMin=[]  SumOutMax=[]  SaturationOutMin=[]  SaturationOutMax=[]  PParamMin=[]  PParamMax=[]  IParamMin=[]  IParamMax=[]  DParamMin=[]  DParamMax=[]  NParamMin=[]  NParamMax=[]  KbParamMin=[]  KbParamMax=[]  KtParamMin=[]  KtParamMax=[]  KbOutMin=[]  KbOutMax=[]  KtOutMin=[]  KtOutMax=[]  IntegratorOutMin=[]  IntegratorOutMax=[]  FilterOutMin=[]  FilterOutMax=[]  SumI1OutMin=[]  SumI1OutMax=[]  SumI2OutMin=[]  SumI2OutMax=[]  SumI3OutMin=[]  SumI3OutMax=[]  SumI4OutMin=[]  SumI4OutMax=[]  SumDOutMin=[]  SumDOutMax=[]  DifferentiatorOutMin=[]  DifferentiatorOutMax=[]  FilterDiffOutCoefMin=[]  FilterDiffOutCoefMax=[]  ReciprocalOutMin=[]  ReciprocalOutMax=[]  SumDenOutMin=[]  SumDenOutMax=[]  SumNumOutMin=[]  SumNumOutMax=[]  DivideOutMin=[]  DivideOutMax=[]  IntegratorContinuousStateAttributes=''  IntegratorStateMustResolveToSignalObject=off  IntegratorRTWStateStorageClass=Auto  FilterContinuousStateAttributes=''  FilterStateMustResolveToSignalObject=off  FilterRTWStateStorageClass=Auto  ParallelPVariant=InternalParameters  IdealPVariant=Disabled  IVariant=InternalParameters  DVariant=Disabled  IntegratorVariant=Discrete  SatVariant=Enabled  AWVariant=Passthrough  PCopyVariant=Disabled  TRVariant=Disabled  FdbkBlocksVariant=Forward  IdealPFdbkVariant=Disabled  SatFdbkVariant=Disabled  DerivativeFilterVariant=Disabled  NVariant=Disabled  NCopyVariant=Disabled_SignalSpec  FilterICVariant=Disabled  IntegratorICVariant=InternalICs  ExternalResetVariant=Disabled  TRSumVariant=Passthrough  SumFdbkVariant=Disabled  SumVariant=Sum_PI
  PI3 : simulink/Continuous/PID Controller  Commented=on  Controller=PI  Form=Parallel  TimeDomain=Discrete-time  SampleTime=Ts_Control  IntegratorMethod=Forward Euler  FilterMethod=Forward Euler  ControllerParametersSource=internal  P=4  I=50  D=0  UseFilter=on  N=100  TunerSelectOption=Transfer Function Based (PID Tuner App)  InitialConditionSource=internal  InitialConditionForIntegrator=0  InitialConditionForFilter=0  DifferentiatorICPrevScaledInput=0  ExternalReset=none  TrackingMode=off  Kt=1  LimitOutput=on  UpperSaturationLimit=90  LowerSaturationLimit=-90  LinearizeAsGain=off  AntiWindupMode=none  Kb=1  POutMin=[]  POutMax=[]  IOutMin=[]  IOutMax=[]  DOutMin=[]  DOutMax=[]  NOutMin=[]  NOutMax=[]  SumOutMin=[]  SumOutMax=[]  SaturationOutMin=[]  SaturationOutMax=[]  PParamMin=[]  PParamMax=[]  IParamMin=[]  IParamMax=[]  DParamMin=[]  DParamMax=[]  NParamMin=[]  NParamMax=[]  KbParamMin=[]  KbParamMax=[]  KtParamMin=[]  KtParamMax=[]  KbOutMin=[]  KbOutMax=[]  KtOutMin=[]  KtOutMax=[]  IntegratorOutMin=[]  IntegratorOutMax=[]  FilterOutMin=[]  FilterOutMax=[]  SumI1OutMin=[]  SumI1OutMax=[]  SumI2OutMin=[]  SumI2OutMax=[]  SumI3OutMin=[]  SumI3OutMax=[]  SumI4OutMin=[]  SumI4OutMax=[]  SumDOutMin=[]  SumDOutMax=[]  DifferentiatorOutMin=[]  DifferentiatorOutMax=[]  FilterDiffOutCoefMin=[]  FilterDiffOutCoefMax=[]  ReciprocalOutMin=[]  ReciprocalOutMax=[]  SumDenOutMin=[]  SumDenOutMax=[]  SumNumOutMin=[]  SumNumOutMax=[]  DivideOutMin=[]  DivideOutMax=[]  IntegratorContinuousStateAttributes=''  IntegratorStateMustResolveToSignalObject=off  IntegratorRTWStateStorageClass=Auto  FilterContinuousStateAttributes=''  FilterStateMustResolveToSignalObject=off  FilterRTWStateStorageClass=Auto  ParallelPVariant=InternalParameters  IdealPVariant=Disabled  IVariant=InternalParameters  DVariant=Disabled  IntegratorVariant=Discrete  SatVariant=Enabled  AWVariant=Passthrough  PCopyVariant=Disabled  TRVariant=Disabled  FdbkBlocksVariant=Forward  IdealPFdbkVariant=Disabled  SatFdbkVariant=Disabled  DerivativeFilterVariant=Disabled  NVariant=Disabled  NCopyVariant=Disabled_SignalSpec  FilterICVariant=Disabled  IntegratorICVariant=InternalICs  ExternalResetVariant=Disabled  TRSumVariant=Passthrough  SumFdbkVariant=Disabled  SumVariant=Sum_PI
  PLL (3ph) : powerlib_meascontrol/PLL/PLL (3ph)  Fmin=55  Par_Init="[-0.57  60]"  ParK=[180, 3200, 1]  TcD=1e-4  MaxRateChangeFreq=12  FilterCutOffFreq=25  Ts=Ts_Power  AGC=on
      settings: SourceProductName=Simscape Electrical
  P_B1 : Scope  NumInputPorts=2
  Power (Positive-Sequence) : powerlib_meascontrol/Measurements/Power (Positive-Sequence)  Freq=60  Vinit=[0, 0]  Iinit=[0, 0]  Ts=Ts_Control
      settings: SourceProductName=Simscape Electrical  SourceProductBaseCode=PS
  Selector : Selector  InputPortWidth=3  IndexOptions=Index vector (dialog)  Indices=[1]  OutputSizes=1
  Selector1 : Selector  InputPortWidth=3  IndexOptions=Index vector (dialog)  Indices=[1]  OutputSizes=1
  Selector2 : Selector  InputPortWidth=3  IndexOptions=Index vector (dialog)  Indices=[1 2]  OutputSizes=1
  Selector3 : Selector  InputPortWidth=3  IndexOptions=Index vector (dialog)  Indices=[1 2]  OutputSizes=1
  Series RLC Branch : powerlib/Elements/Series RLC Branch  Commented=on  LConnTagsString=__new0  RConnTagsString=__new0  BranchType=L  Resistance=1  Inductance=1.5e-6  SetiL0=off  InitialCurrent=0  Capacitance=1e-6  Setx0=off  InitialVoltage=0  Measurements=None
      settings: SourceProductName=Simscape Electrical
  Series RLC Branch1 : powerlib/Elements/Series RLC Branch  Commented=on  LConnTagsString=__new0  RConnTagsString=__new0  BranchType=R  Resistance=3.2  Inductance=1e-3  SetiL0=off  InitialCurrent=0  Capacitance=1200e-6  Setx0=off  InitialVoltage=400  Measurements=None
      settings: SourceProductName=Simscape Electrical
  Series RLC Branch4 : powerlib/Elements/Series RLC Branch  LConnTagsString=__new0  RConnTagsString=__new0  BranchType=RC  Resistance=1e-7  Inductance=1e-3  SetiL0=off  InitialCurrent=0  Capacitance=3600e-6  Setx0=off  InitialVoltage=400  Measurements=None
      settings: SourceProductName=Simscape Electrical
  Subsystem : Subsystem  Commented=on
  Sum : Sum  Inputs=|-+
  Sum3 : Sum  Commented=on  Inputs=|-+
  Terminator : Terminator
  Terminator1 : Terminator
  Three-Phase Breaker : powerlib/Elements/Three-Phase Breaker  InitialState=open  SwitchA=on  SwitchB=on  SwitchC=on  SwitchTimes="[1/6  5/6]"  External=on  BreakerResistance=0.01e-3  SnubberResistance=30  SnubberCapacitance=20e-6  Measurements=None
      settings: SourceProductName=Simscape Electrical
  VSC (Average Model) : powerlib/Power Electronics/Universal Bridge  Arms=3  SnubberResistance=1e5  SnubberCapacitance=inf  Device=Average-model based VSC  Ron=1e-3  Lon=0  ForwardVoltages="[  0  0  ]"  ForwardVoltage=0  GTOparameters=[ 10e-6 , 20e-6 ]  IGBTparameters=[ 1e-6 , 2e-6 ]  Measurements=None  Measurements_2=None  converterType=Rectifier
      settings: SourceProductName=Simscape Electrical
  VSC (Average Model)1 : powerlib/Power Electronics/Universal Bridge  Commented=on  Arms=2  SnubberResistance=1e5  SnubberCapacitance=inf  Device=Average-model based VSC  Ron=1e-3  Lon=0  ForwardVoltages="[  0  0  ]"  ForwardVoltage=0  GTOparameters=[ 10e-6 , 20e-6 ]  IGBTparameters=[ 1e-6 , 2e-6 ]  Measurements=None  Measurements_2=None  converterType=Rectifier
      settings: SourceProductName=Simscape Electrical
  VSC (Average Model)2 : powerlib/Power Electronics/Universal Bridge  Commented=on  Arms=2  SnubberResistance=1e5  SnubberCapacitance=inf  Device=Average-model based VSC  Ron=1e-3  Lon=0  ForwardVoltages="[  0  0  ]"  ForwardVoltage=0  GTOparameters=[ 10e-6 , 20e-6 ]  IGBTparameters=[ 1e-6 , 2e-6 ]  Measurements=None  Measurements_2=None  converterType=Rectifier
      settings: SourceProductName=Simscape Electrical
  V_I grid : Scope  NumInputPorts=2
  Vdc_bus1 : Scope
  Voltage Measurement1 : powerlib/Measurements/Voltage Measurement  PhasorSimulation=off  OutputType=Complex  PSBequivalent=0
      settings: SourceProductName=Simscape Electrical
  W2kW : Gain  Gain=1/1000
  W2kW1 : Gain  Gain=1/1000
  abc to dq0 : powerlib_meascontrol/Transformations/abc to dq0  Alignment=90 degrees behind phase A axis
      settings: SourceProductName=Simscape Electrical
  abc to dq1 : powerlib_meascontrol/Transformations/abc to dq0  Alignment=90 degrees behind phase A axis
      settings: SourceProductName=Simscape Electrical
  dq0 to abc : powerlib_meascontrol/Transformations/dq0 to abc  Alignment=90 degrees behind phase A axis
      settings: SourceProductName=Simscape Electrical
  a : PMIOPort  Side=Right
  b : PMIOPort  Port=2  Side=Right
  c : PMIOPort  Port=3  Side=Right
  Out1 : Outport
  Qcap : Outport  Port=2
  Pcap : Outport  Port=3
  wires:
  PLL (3ph)/2 -> abc to dq1/2, abc to dq0/2, dq0 to abc/2
  Subsystem/1(Uref_DAB1) -> VSC (Average Model)2/1
  PI/1 -> Mux3/1
  Selector/1 -> V_I grid/1  "Va (V)"
  dq0 to abc/1 -> Gain/1
  Vdc_bus_ref/1 -> Sum3/2
  PLL (3ph)/1 -> Terminator/1
  [Iabc_B1_EV5] -> Selector1/1, Power (Positive-Sequence)/2
  abc to dq1/1 -> Selector2/1
  Mux3/1 -> dq0 to abc/1
  Gain/1 -> VSC (Average Model)/1
  W2kW1/1 -> P_B1/2  "Q (kVA)"
  Selector2/1 -> Sum/1
  Sum/1 -> PI/1
  [Vabc_B2_EV5] -> abc to dq0/1, PLL (3ph)/1
  Subsystem/2(Uref_DAB2) -> VSC (Average Model)1/1
  Sum3/1 -> PI3/1
  W2kW/1 -> P_B1/1  "P (kW)"
  Constant2/1 -> Mux3/2
  PI3/1 -> Subsystem/1(phase shift (-90,90))
  Selector3/1 -> Demux/1
  [Vabc_B2_EV5] -> Selector/1, Power (Positive-Sequence)/1
  Selector1/1 -> V_I grid/2
  From4/1 -> Sum3/1
  abc to dq0/1 -> Selector3/1
  Power (Positive-Sequence)/1 -> W2kW/1
  Voltage Measurement1/1 -> Vdc_bus1/1, [Vdc_EV5]
  Mux2/1 -> Sum/2
  [Iabc_B1_EV5] -> abc to dq1/1
  Power (Positive-Sequence)/2 -> W2kW1/1
  Battery/1 -> Out1/1  "Battery"
  on-off breaker/1 -> Three-Phase Breaker/1
  Demux/2 -> Terminator1/1
  Demux/1 -> [Vd_EV5]
  MATLAB Function/1(id) -> Mux2/1
  MATLAB Function/2(iq) -> Mux2/2
  [Vd_EV5] -> MATLAB Function/3(vd)
  P/1 -> MATLAB Function/1(P)  "P"
  Q/1 -> MATLAB Function/2(Q)  "Q"
  Constant/1 -> Qcap/1
  Constant1/1 -> Pcap/1
  connections:
  Battery/LConn1 -- VSC (Average Model)1/RConn1
  Three-Phase Breaker/LConn1 -- B1/RConn1
  Three-Phase Breaker/RConn2 -- B2/LConn2
  VSC (Average Model)/RConn2 -- Series RLC Branch1/RConn1 -- Voltage Measurement1/LConn2 -- DC Voltage Source/LConn1 -- Series RLC Branch4/RConn1 -- VSC (Average Model)2/RConn2
  L/RConn3 -- B1/LConn3
  L/LConn1 -- VSC (Average Model)/LConn1
  L/RConn1 -- B1/LConn1
  L/LConn2 -- VSC (Average Model)/LConn2
  Series RLC Branch1/LConn1 -- VSC (Average Model)/RConn1 -- DC Voltage Source/RConn1 -- VSC (Average Model)2/RConn1 -- Series RLC Branch4/LConn1 -- Voltage Measurement1/LConn1
  Series RLC Branch/RConn1 -- Linear Transformer/LConn1
  Linear Transformer/LConn2 -- VSC (Average Model)1/LConn2
  Three-Phase Breaker/LConn2 -- B1/RConn2
  VSC (Average Model)1/RConn2 -- Battery/LConn2
  Three-Phase Breaker/RConn3 -- B2/LConn3
  Three-Phase Breaker/RConn1 -- B2/LConn1
  Linear Transformer/RConn1 -- VSC (Average Model)2/LConn1
  Linear Transformer/RConn2 -- VSC (Average Model)2/LConn2
  c/RConn1 -- B2/RConn3
  Series RLC Branch/LConn1 -- VSC (Average Model)1/LConn1
  L/RConn2 -- B1/LConn2
  L/LConn3 -- VSC (Average Model)/LConn3
  Three-Phase Breaker/LConn3 -- B1/RConn3
  b/RConn1 -- B2/RConn2
  a/RConn1 -- B2/RConn1
